simulink model "ami"  (R2015b)
settings: Solver=VariableStepAuto  StartTime=0.0  StopTime=2  RelTol=1e-3
settings Model: Creator=ovi  LastModifiedBy=ovi

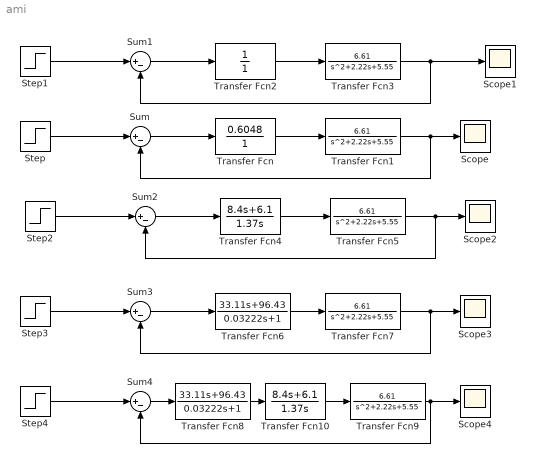
== system ami ==
  Scope{,1..4} (5 alike) : Scope
  Step : Step  SampleTime=0
  Step1 : Step  SampleTime=0
  Step2 : Step  SampleTime=0
  Step3 : Step  Time=0.5  SampleTime=0
  Step4 : Step  Time=0.5  SampleTime=0
  Sum{,1..4} (5 alike) : Sum  Inputs=|+-
  Transfer Fcn : TransferFcn  Numerator=[0.6048]  Denominator=[1]
  Transfer Fcn{1,3,5,7,9} (5 alike) : TransferFcn  Numerator=[6.61]  Denominator=[1 2.22 5.55]
  Transfer Fcn10 : TransferFcn  Numerator=[8.4 6.1]  Denominator=[1.37 0]
  Transfer Fcn2 : TransferFcn  Denominator=[1]
  Transfer Fcn4 : TransferFcn  Numerator=[8.4 6.1]  Denominator=[1.37 0]
  Transfer Fcn6 : TransferFcn  Numerator=[33.11 96.43]  Denominator=[0.03222 1]
  Transfer Fcn8 : TransferFcn  Numerator=[33.11 96.43]  Denominator=[0.03222 1]
  wires:
  Transfer Fcn/1 -> Transfer Fcn1/1
  Step/1 -> Sum/1
  Sum/1 -> Transfer Fcn/1
  Transfer Fcn1/1 -> Sum/2, Scope/1
  Transfer Fcn2/1 -> Transfer Fcn3/1
  Step1/1 -> Sum1/1
  Sum1/1 -> Transfer Fcn2/1
  Transfer Fcn3/1 -> Sum1/2, Scope1/1
  Transfer Fcn4/1 -> Transfer Fcn5/1
  Step2/1 -> Sum2/1
  Sum2/1 -> Transfer Fcn4/1
  Transfer Fcn5/1 -> Sum2/2, Scope2/1
  Transfer Fcn6/1 -> Transfer Fcn7/1
  Step3/1 -> Sum3/1
  Sum3/1 -> Transfer Fcn6/1
  Transfer Fcn7/1 -> Sum3/2, Scope3/1
  Transfer Fcn8/1 -> Transfer Fcn10/1
  Step4/1 -> Sum4/1
  Sum4/1 -> Transfer Fcn8/1
  Transfer Fcn9/1 -> Sum4/2, Scope4/1
  Transfer Fcn10/1 -> Transfer Fcn9/1
